simulink model "block_vrml"  (R2019a)
settings: Solver=VariableStepAuto  StartTime=0.0  StopTime=10.0  RelTol=1e-3
libraries: vrlib x2
settings Model: Creator=Imanol  LastModifiedBy=Imanol

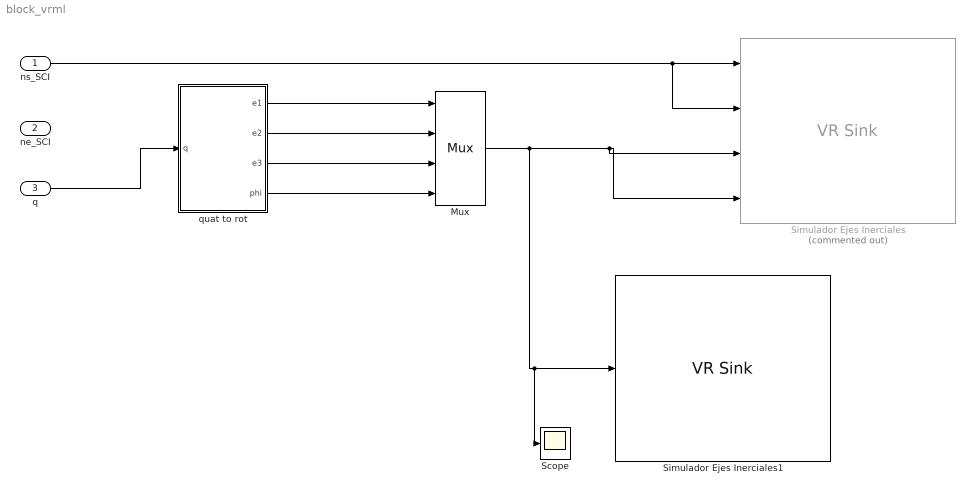
== system block_vrml ==
  ns_SCI : Inport  PortDimensions=[3,1]
  ne_SCI : Inport  Port=2  PortDimensions=[3,1]
  q : Inport  Port=3  PortDimensions=[4,1]
  Mux : Mux
  Scope : Scope
  Simulador Ejes Inerciales : vrlib/VR Sink  Commented=on  InstantiateOnLoad=on  SampleTime=1e-2  ViewEnable=on  RemoteChange=off  RemoteView=off  FieldsWritten=Light_transform.translation.3.1.1.double#SunVectorPosition.translation.3.1.1.double#BodyCoor.rotation.4.1.1.double#Cubasat_transform.rotation.4.1.1.double  WorldFileName=myworld.wrl  AutoView=off  VideoDimensions=[]  AllowVariableSize=off
      settings: SourceProductBaseCode=VR
  Simulador Ejes Inerciales1 : vrlib/VR Sink  InstantiateOnLoad=on  SampleTime=1e-2  ViewEnable=on  RemoteChange=off  RemoteView=on  FieldsWritten=BodyCoor.rotation.4.1.1.double  WorldFileName=myworldV2.wrl  AutoView=off  VideoDimensions=[]  AllowVariableSize=off
      settings: SourceProductBaseCode=VR
  quat to rot : MATLAB Function  TreatAsAtomicUnit=on
  wires:
  q/1 -> quat to rot/1(q)
  quat to rot/2(e2) -> Mux/2
  quat to rot/1(e1) -> Mux/1
  quat to rot/3(e3) -> Mux/3
  quat to rot/4(phi) -> Mux/4
  ns_SCI/1 -> Simulador Ejes Inerciales/2, Simulador Ejes Inerciales/1
  Mux/1 -> Scope/1, Simulador Ejes Inerciales1/1, Simulador Ejes Inerciales/3, Simulador Ejes Inerciales/4

== matlab function block_vrml/quat to rot ==
  data: e1 output; q input; e2 output; e3 output; phi output
function [e1, e2, e3, phi] = fcn(q)
ee2 = zeros(3, 1);
ee2(1) = q(1);
ee2(2) = q(2);
ee2(3) = q(3);
c_half = q(4);
if abs(abs(c_half) - 1e0) < 1e-5
    phi = 2e0 * acos(c_half) * 180e0 / pi;
    e1 = 1e0;
    e2 = 0e0;
    e3 = 0e0;
else
    s2_half = dot(ee2, ee2);
    s_half = sqrt(s2_half);
    phi = 2e0 * atan2(s_half, c_half) * 180. / pi;
    e1 = ee2(1) / s_half;
    e2 = ee2(2) / s_half;
    e3 = ee2(3) / s_half;
end
% e = ee2 / norm(ee2);
% if (norm(e) < 1e-5)
%   phi = 0e0;
% else
%   if(abs(e(1)) > 1e-5)
%     s_half = ee2(1) / e(1);
%   elseif (abs(e(1)) > 1e-5)
%     s_half = ee2(2) / e(2);
%   else
%     s_half = ee2(3) / e(3);
%   end
%   phi = 2e0 * atan2(s_half, q(4));
% end
% %s = maxval(e2(abs(e2) > 1e-5) ./ e(abs(e2) > 1e-5));
% % phi = 2e0 * atan2(s, qq(4)) * 180. / pi;
% e1 = e(1);
% e2 = e(2);
% e3 = e(3);
% %phi = phi;
% 
% %q1 = qq(1);
% %q2 = qq(2);
% %q3 = qq(3);
% %q4 = qq(4);
